simulink model "Problem_6"  (R2020a)
settings: Solver=VariableStepAuto  StartTime=0.0  StopTime=10.0  RelTol=1e-3
settings Model: Creator=Saqlain  LastModifiedBy=Saqlain

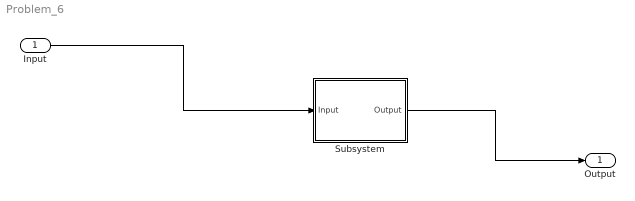
== system Problem_6 ==
  Input : Inport
  Subsystem : Subsystem
  Output : Outport
  wires:
  Input/1 -> Subsystem/1(Input)
  Subsystem/1(Output) -> Output/1

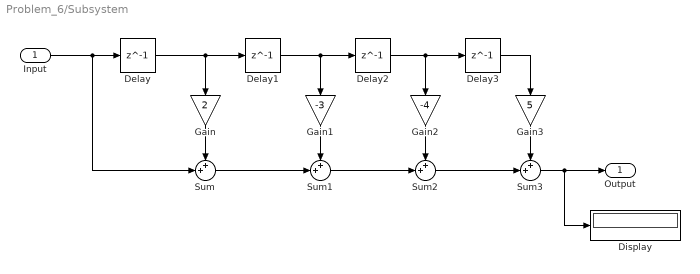
== system Problem_6/Subsystem ==
  Input : Inport
  Delay{,1..3} (4 alike) : Delay  DelayLength=1
  Display : Display
  Gain : Gain  Gain=2
  Gain1 : Gain  Gain=-3
  Gain2 : Gain  Gain=-4
  Gain3 : Gain  Gain=5
  Sum{,1..3} (4 alike) : Sum  Inputs=++|
  Output : Outport
  wires:
  Delay1/1 -> Gain1/1, Delay2/1
  Sum/1 -> Sum1/2
  Delay2/1 -> Gain2/1, Delay3/1
  Sum1/1 -> Sum2/2
  Input/1 -> Sum/2, Delay/1
  Sum2/1 -> Sum3/2
  Delay3/1 -> Gain3/1
  Gain/1 -> Sum/1
  Delay/1 -> Gain/1, Delay1/1
  Gain2/1 -> Sum2/1
  Sum3/1 -> Output/1, Display/1
  Gain3/1 -> Sum3/1
  Gain1/1 -> Sum1/1
